simulink model "lab4s"  (R2024b)
settings: Solver=VariableStepAuto  StartTime=0.0  StopTime=10.0  MaxStep=0.1  RelTol=1e-3
values from neighbouring files (symbols this model uses):
  czas_skok = 20    [lab4.m]
  dU = 0    [lab4.m]
  ksi = -0.75    [lab4.m]
  omega_n = 0.5    [lab4.m]
  U0 = 0    [lab4.m]
  x0 = U0    (= 0)    [lab4.m]
  x_prim0 = tabl_x_prim0(i)    [lab4.m]
settings Model: Creator=Adam  LastModifiedBy=Adam

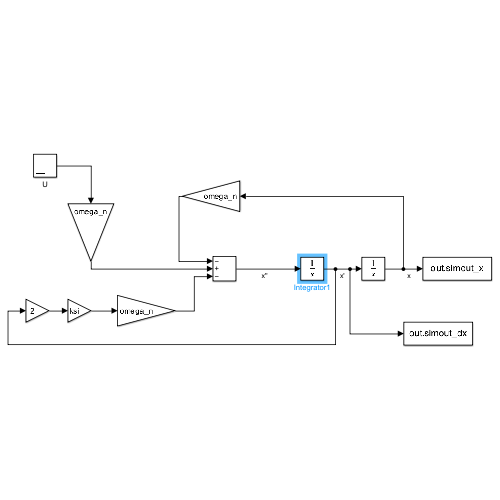
[thumbnail: Simulink's stored preview of the top-level diagram]
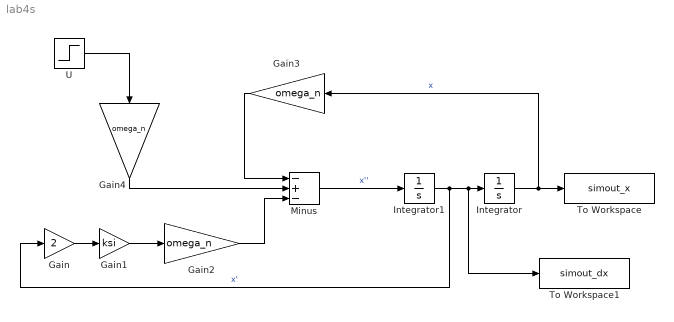
== system lab4s ==
  Gain : Gain  Gain=2
  Gain1 : Gain  Gain=ksi
  Gain2 : Gain  Gain=omega_n
  Gain3 : Gain  Gain=omega_n
  Gain4 : Gain  Gain=omega_n
  Integrator : Integrator  InitialCondition=x0
  Integrator1 : Integrator  InitialCondition=x_prim0
  Minus : Sum  Inputs=-+-
  To Workspace : ToWorkspace  VariableName=simout_x  SampleTime=-1
  To Workspace1 : ToWorkspace  VariableName=simout_dx  SampleTime=-1
  U : Step  Time=czas_skok  Before=U0  After=U0+dU  SampleTime=0
  wires:
  Integrator1/1 -> Gain/1, To Workspace1/1, Integrator/1  "x'"
  Gain/1 -> Gain1/1
  Gain1/1 -> Gain2/1
  Minus/1 -> Integrator1/1  "x''"
  Integrator/1 -> Gain3/1, To Workspace/1  "x"
  Gain3/1 -> Minus/1
  Gain2/1 -> Minus/3
  Gain4/1 -> Minus/2
  U/1 -> Gain4/1
